simulink model "M4B11_modified_AGC_PI"  (R2025a)
settings: Solver=VariableStepAuto  StartTime=0.0  StopTime=100  RelTol=1e-3
InitFcn:
  | clear;
  | load('parameterinit.mat');
  | set_param('M4B11_modified_AGC_PI/Python2Sim','value','[0 0 0 0 0 0 0 0]');
  | acom=100;
  | bcom=50;
  | lam=100;
values from neighbouring files (symbols this model uses):
  ACgirdinit =     [datainit.mat]    (also in parameterinit.mat)
  AVm0 = [11.3576294988 11.3576294988]    [datainit.mat]    (also in parameterinit.mat)
  commun = [1 1 1 0]    [datainit.mat]    (also in initAll.m = [1,1,1,0]; parameterinit.mat)
  DataDelay = [0  0; 0  0; 0  0; 0  0]    [datainit.mat]    (also in initAll.m = 0.0*DataDelay; parameterinit.mat)
  ESinit =     [datainit.mat]    (also in parameterinit.mat)
  fB = 50    [datainit.mat]    (also in initAll.m; parameterinit.mat)
  Geninit =     [datainit.mat]    (also in initAll.m = Generator_init(opdata,SynMach_in_gidx); parameterinit.mat)
  SgridB = 100    [datainit.mat]    (also in initAll.m = resultsac.baseMVA; parameterinit.mat)
  wB = 314.159265359    [datainit.mat]    (also in initAll.m; parameterinit.mat)
  Windinit =     [datainit.mat]    (also in parameterinit.mat)
undefined symbols (not defined in the file or in its folder): c1, c2, c3, c4, c5, c6, cp_nom, lambda_nom, P_wind_base, Pelec_base, Pnom
libraries: spsBistableLib x9, slpidlib x2, simulink_extras x2
(part 1 of 6)
settings Model: Creator=LinSiQi  LastModifiedBy=86182
settings SolverCC: AlgebraicLoopSolver=TrustRegion
settings DataIOCC: DSMLogging=off  ReturnWorkspaceOutputs=off  SignalLoggingName=logout
settings DebuggingCC: UnconnectedInputMsg=warning  UnconnectedOutputMsg=warning  UnconnectedLineMsg=warning  ArithmeticOperatorsInVariantConditions=warning
settings ModelReferenceCC: EnableRefExpFcnMdlSchedulingChecks=on
settings SFSimCC: CustomCodeUndefinedFunction=UseInterfaceOnly
settings RTWCC: GPUComputeCapability=3.5  DLArmComputeVersion=19.05
settings CodeAppCC: StateflowObjectComments=on
settings SimscapeCC: SimscapeNormalizeSystem=off

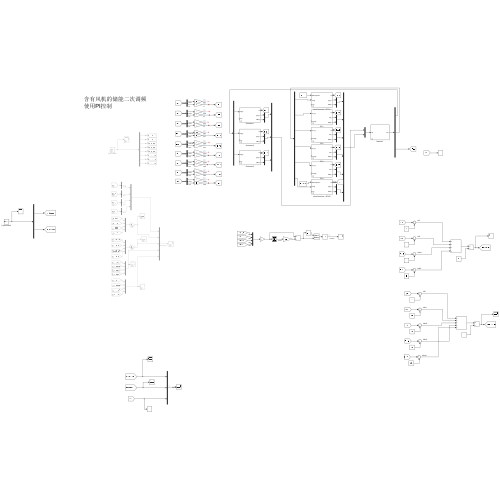
[thumbnail: Simulink's stored preview of the top-level diagram]
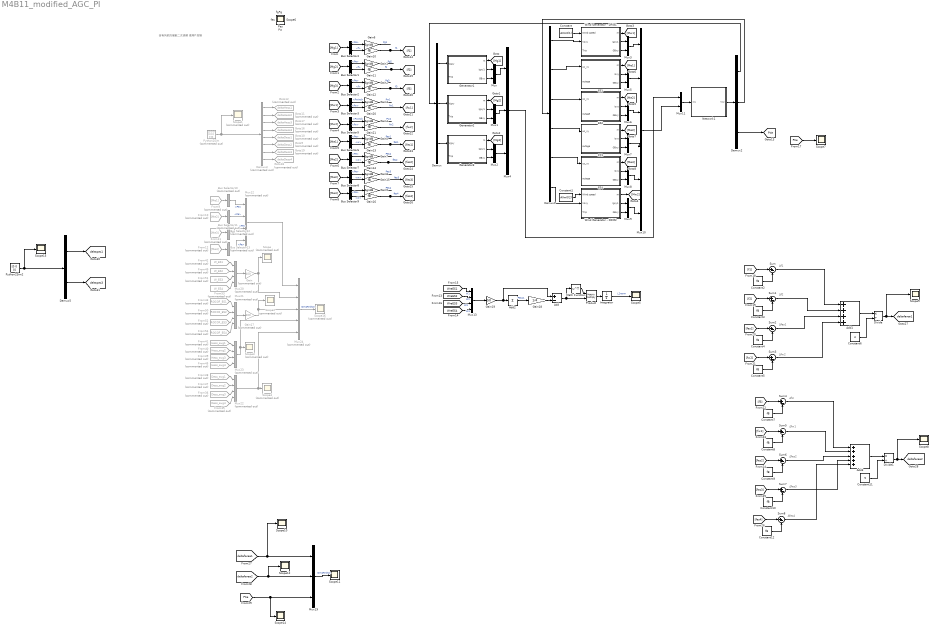
== system M4B11_modified_AGC_PI ==
  note: 含有风机的储能二次调频
      | 使用PI控制
  note: Δf1
  note: Δf2
  note: Δfes1
  note: Δfw2
  note: Δf3
  note: Δfes2
  note: Δfes3
  note: Δfw1
  note: Δfes4
  Add : Sum  Inputs=+-
  Add1 : Sum  Inputs=++++
  Add2 : Sum  Inputs=+
  Add3 : Sum  Inputs=+++++
  Bus Selector1 : BusSelector  OutputSignals=Pe,f
  Bus Selector{10..13} (4 alike) : BusSelector  Commented=on  OutputSignals=Pe
  Bus Selector2 : BusSelector  OutputSignals=Pe,f
  Bus Selector3 : BusSelector  OutputSignals=Pwind,fw
  Bus Selector4 : BusSelector  OutputSignals=Pe,f
  Bus Selector5 : BusSelector  OutputSignals=Pwind,fw
  Bus Selector{6..9} (4 alike) : BusSelector  OutputSignals=Pe,w
  Constant : Constant  Value=AVm0(1)
  Constant1 : Constant  Value=AVm0(2)
  Constant{2..5,7..10,12} (9 alike) : Constant  Value=fB
  Constant11 : Constant  Value=5
  Constant6 : Constant  Value=4
  Demux : Demux  Outputs=3
  Demux1 : Demux  Outputs=6
  Demux2 : Demux  Outputs=[6 12 1]
  Demux3 : Demux  Commented=on  Outputs=8
  Demux5 : Demux  Outputs=2
  Divide : Product  Inputs=*/
  Divide1 : Product  Inputs=*/
  ES1 : Subsystem  mask{SvscB=ESinit.SvscBi(1), SgridB=SgridB, Kppll_VSC=ESinit.Kppll(1), Kipll_VSC=ESinit.Kipll(1), Dels_hvdc=ESinit.Dels_hvdc(1), Lpr=ESinit.Lpr(1), Rpr=ESinit.Rpr(1), wB=wB, Is_xA_0=ESinit.Isx0(1), Is_yA_0=ESinit.Isy0(1), KpP_VSC_A=ESinit.KpP(1), KiP_VSC_A=ESinit.KiP(1), KpId_VSC_A=ESinit.KpId(1), KiId_VSC_A=ESinit.KiId(1), KpQ_VSC_A=ESinit.KpQ(1), KiQ_VSC_A=ESinit.KiQ(1), KpIq_VSC_A=ESinit.KpIq(1), KiIq_VSC_A=ESinit.KiIq(1), Md_A_0=ESinit.Md0(1), Mq_A_0=ESinit.Mq0(1), Nd_A_0=ESinit.Nd0(1), Nq_A_0=ESinit.Nq0(1), KIR=ESinit.Kir(1), Kdroop=ESinit.Kdroop(1), Kdistributed=ESinit.Kdistributed(1), Kdistributed_d=ESinit.Kdistributed_d(1), Kpac_VSC_A=ESinit.Kpac(1), Kiac_VSC_A=ESinit.Kiac(1), P0=ESinit.P0(1), Q0=ESinit.Q0(1), usd0=ESinit.Usd0(1)}
      mask prompts: Kppll_VSC "Kppll"; Kipll_VSC "Kipll"; KpP_VSC_A "KpP"; KiP_VSC_A "KiP"; KpId_VSC_A "KpId"; KiId_VSC_A "KiId"; KpQ_VSC_A "KpQ"; KiQ_VSC_A "KiQ"; KpIq_VSC_A "KpIq"; KiIq_VSC_A "KiIq"; Kpac_VSC_A "Kpac"; Kiac_VSC_A "Kiac"
      mask DialogControl Container48 Prompt: Base value
      mask DialogControl Container7 Prompt: PLL
      mask DialogControl Container5 Prompt: Control parameter
      mask DialogControl Container8 Prompt: inital value
      mask DialogControl Container9 Prompt: AC side
      mask DialogControl Container10 Prompt: Parameter
      mask DialogControl Container11 Prompt: Initial value
      mask DialogControl Container18 Prompt: Control parameter
      mask DialogControl Container19 Prompt: d_axis_control parameter
      mask DialogControl Container23 Prompt: d_axis_control=1
      mask DialogControl Container26 Prompt: inner current control
      mask DialogControl Container21 Prompt: q_axis_control parameter
      mask DialogControl Container29 Prompt: q_axis_control=1
      mask DialogControl Container31 Prompt: inner current control
      mask DialogControl Container22 Prompt: inital value
      mask DialogControl Container35 Prompt: outer controller
      mask DialogControl Container36 Prompt: inner control
      mask DialogControl Container27 Prompt: Inertia control
      mask DialogControl Container28 Prompt: droop control
      mask DialogControl Container300 Prompt: distributed control
      mask DialogControl Container301 Prompt: Droop distributed control
      mask DialogControl Container40 Prompt: usdq_control
      mask DialogControl Container41 Prompt: PQinitial
      mask DialogControl Container42 Prompt: usd0initial
  ES2 : Subsystem  mask{SvscB=ESinit.SvscBi(2), SgridB=SgridB, Kppll_VSC=ESinit.Kppll(2), Kipll_VSC=ESinit.Kipll(2), Dels_hvdc=ESinit.Dels_hvdc(2), Lpr=ESinit.Lpr(2), Rpr=ESinit.Rpr(2), wB=wB, Is_xA_0=ESinit.Isx0(2), Is_yA_0=ESinit.Isy0(2), KpP_VSC_A=ESinit.KpP(2), KiP_VSC_A=ESinit.KiP(2), KpId_VSC_A=ESinit.KpId(2), KiId_VSC_A=ESinit.KiId(2), KpQ_VSC_A=ESinit.KpQ(2), KiQ_VSC_A=ESinit.KiQ(2), KpIq_VSC_A=ESinit.KpIq(2), KiIq_VSC_A=ESinit.KiIq(2), Md_A_0=ESinit.Md0(2), Mq_A_0=ESinit.Mq0(2), Nd_A_0=ESinit.Nd0(2), Nq_A_0=ESinit.Nq0(2), KIR=ESinit.Kir(2), Kdroop=ESinit.Kdroop(2), Kdistributed=ESinit.Kdistributed(2), Kdistributed_d=ESinit.Kdistributed_d(2), Kpac_VSC_A=ESinit.Kpac(2), Kiac_VSC_A=ESinit.Kiac(2), P0=ESinit.P0(2), Q0=ESinit.Q0(2), usd0=ESinit.Usd0(2)}
      mask prompts: Kppll_VSC "Kppll"; Kipll_VSC "Kipll"; KpP_VSC_A "KpP"; KiP_VSC_A "KiP"; KpId_VSC_A "KpId"; KiId_VSC_A "KiId"; KpQ_VSC_A "KpQ"; KiQ_VSC_A "KiQ"; KpIq_VSC_A "KpIq"; KiIq_VSC_A "KiIq"; Kpac_VSC_A "Kpac"; Kiac_VSC_A "Kiac"
      mask DialogControl Container48 Prompt: Base value
      mask DialogControl Container7 Prompt: PLL
      mask DialogControl Container5 Prompt: Control parameter
      mask DialogControl Container8 Prompt: inital value
      mask DialogControl Container9 Prompt: AC side
      mask DialogControl Container10 Prompt: Parameter
      mask DialogControl Container11 Prompt: Initial value
      mask DialogControl Container18 Prompt: Control parameter
      mask DialogControl Container19 Prompt: d_axis_control parameter
      mask DialogControl Container23 Prompt: d_axis_control=1
      mask DialogControl Container26 Prompt: inner current control
      mask DialogControl Container21 Prompt: q_axis_control parameter
      mask DialogControl Container29 Prompt: q_axis_control=1
      mask DialogControl Container31 Prompt: inner current control
      mask DialogControl Container22 Prompt: inital value
      mask DialogControl Container35 Prompt: outer controller
      mask DialogControl Container36 Prompt: inner control
      mask DialogControl Container27 Prompt: Inertia control
      mask DialogControl Container28 Prompt: droop control
      mask DialogControl Container300 Prompt: distributed control
      mask DialogControl Container301 Prompt: Droop distributed control
      mask DialogControl Container40 Prompt: usdq_control
      mask DialogControl Container41 Prompt: PQinitial
      mask DialogControl Container42 Prompt: usd0initial
  ES3 : Subsystem  mask{SvscB=ESinit.SvscBi(3), SgridB=SgridB, Kppll_VSC=ESinit.Kppll(3), Kipll_VSC=ESinit.Kipll(3), Dels_hvdc=ESinit.Dels_hvdc(3), Lpr=ESinit.Lpr(3), Rpr=ESinit.Rpr(3), wB=wB, Is_xA_0=ESinit.Isx0(3), Is_yA_0=ESinit.Isy0(3), KpP_VSC_A=ESinit.KpP(3), KiP_VSC_A=ESinit.KiP(3), KpId_VSC_A=ESinit.KpId(3), KiId_VSC_A=ESinit.KiId(3), KpQ_VSC_A=ESinit.KpQ(3), KiQ_VSC_A=ESinit.KiQ(3), KpIq_VSC_A=ESinit.KpIq(3), KiIq_VSC_A=ESinit.KiIq(3), Md_A_0=ESinit.Md0(3), Mq_A_0=ESinit.Mq0(3), Nd_A_0=ESinit.Nd0(3), Nq_A_0=ESinit.Nq0(3), KIR=ESinit.Kir(3), Kdroop=ESinit.Kdroop(3), Kdistributed=ESinit.Kdistributed(3), Kdistributed_d=ESinit.Kdistributed_d(3), Kpac_VSC_A=ESinit.Kpac(3), Kiac_VSC_A=ESinit.Kiac(3), P0=ESinit.P0(3), Q0=ESinit.Q0(3), usd0=ESinit.Usd0(3)}
      mask prompts: Kppll_VSC "Kppll"; Kipll_VSC "Kipll"; KpP_VSC_A "KpP"; KiP_VSC_A "KiP"; KpId_VSC_A "KpId"; KiId_VSC_A "KiId"; KpQ_VSC_A "KpQ"; KiQ_VSC_A "KiQ"; KpIq_VSC_A "KpIq"; KiIq_VSC_A "KiIq"; Kpac_VSC_A "Kpac"; Kiac_VSC_A "Kiac"
      mask DialogControl Container48 Prompt: Base value
      mask DialogControl Container7 Prompt: PLL
      mask DialogControl Container5 Prompt: Control parameter
      mask DialogControl Container8 Prompt: inital value
      mask DialogControl Container9 Prompt: AC side
      mask DialogControl Container10 Prompt: Parameter
      mask DialogControl Container11 Prompt: Initial value
      mask DialogControl Container18 Prompt: Control parameter
      mask DialogControl Container19 Prompt: d_axis_control parameter
      mask DialogControl Container23 Prompt: d_axis_control=1
      mask DialogControl Container26 Prompt: inner current control
      mask DialogControl Container21 Prompt: q_axis_control parameter
      mask DialogControl Container29 Prompt: q_axis_control=1
      mask DialogControl Container31 Prompt: inner current control
      mask DialogControl Container22 Prompt: inital value
      mask DialogControl Container35 Prompt: outer controller
      mask DialogControl Container36 Prompt: inner control
      mask DialogControl Container27 Prompt: Inertia control
      mask DialogControl Container28 Prompt: droop control
      mask DialogControl Container300 Prompt: distributed control
      mask DialogControl Container301 Prompt: Droop distributed control
      mask DialogControl Container40 Prompt: usdq_control
      mask DialogControl Container41 Prompt: PQinitial
      mask DialogControl Container42 Prompt: usd0initial
  ES4 : Subsystem  mask{SvscB=ESinit.SvscBi(4), SgridB=SgridB, Kppll_VSC=ESinit.Kppll(4), Kipll_VSC=ESinit.Kipll(4), Dels_hvdc=ESinit.Dels_hvdc(4), Lpr=ESinit.Lpr(4), Rpr=ESinit.Rpr(4), wB=wB, Is_xA_0=ESinit.Isx0(4), Is_yA_0=ESinit.Isy0(4), KpP_VSC_A=ESinit.KpP(4), KiP_VSC_A=ESinit.KiP(4), KpId_VSC_A=ESinit.KpId(4), KiId_VSC_A=ESinit.KiId(4), KpQ_VSC_A=ESinit.KpQ(4), KiQ_VSC_A=ESinit.KiQ(4), KpIq_VSC_A=ESinit.KpIq(4), KiIq_VSC_A=ESinit.KiIq(4), Md_A_0=ESinit.Md0(4), Mq_A_0=ESinit.Mq0(4), Nd_A_0=ESinit.Nd0(4), Nq_A_0=ESinit.Nq0(4), KIR=ESinit.Kir(4), Kdroop=ESinit.Kdroop(4), Kdistributed=ESinit.Kdistributed(4), Kdistributed_d=ESinit.Kdistributed_d(4), Kpac_VSC_A=ESinit.Kpac(4), Kiac_VSC_A=ESinit.Kiac(4), P0=ESinit.P0(4), Q0=ESinit.Q0(4), usd0=ESinit.Usd0(4)}
      mask prompts: Kppll_VSC "Kppll"; Kipll_VSC "Kipll"; KpP_VSC_A "KpP"; KiP_VSC_A "KiP"; KpId_VSC_A "KpId"; KiId_VSC_A "KiId"; KpQ_VSC_A "KpQ"; KiQ_VSC_A "KiQ"; KpIq_VSC_A "KpIq"; KiIq_VSC_A "KiIq"; Kpac_VSC_A "Kpac"; Kiac_VSC_A "Kiac"
      mask DialogControl Container48 Prompt: Base value
      mask DialogControl Container7 Prompt: PLL
      mask DialogControl Container5 Prompt: Control parameter
      mask DialogControl Container8 Prompt: inital value
      mask DialogControl Container9 Prompt: AC side
      mask DialogControl Container10 Prompt: Parameter
      mask DialogControl Container11 Prompt: Initial value
      mask DialogControl Container18 Prompt: Control parameter
      mask DialogControl Container19 Prompt: d_axis_control parameter
      mask DialogControl Container23 Prompt: d_axis_control=1
      mask DialogControl Container26 Prompt: inner current control
      mask DialogControl Container21 Prompt: q_axis_control parameter
      mask DialogControl Container29 Prompt: q_axis_control=1
      mask DialogControl Container31 Prompt: inner current control
      mask DialogControl Container22 Prompt: inital value
      mask DialogControl Container35 Prompt: outer controller
      mask DialogControl Container36 Prompt: inner control
      mask DialogControl Container27 Prompt: Inertia control
      mask DialogControl Container28 Prompt: droop control
      mask DialogControl Container300 Prompt: distributed control
      mask DialogControl Container301 Prompt: Droop distributed control
      mask DialogControl Container40 Prompt: usdq_control
      mask DialogControl Container41 Prompt: PQinitial
      mask DialogControl Container42 Prompt: usd0initial
  From10 : From  Commented=on  GotoTag=Me2
  From11 : From  Commented=on  GotoTag=Me3
  From12 : From  Commented=on  GotoTag=Me4
  From35 : From  Commented=on  GotoTag=Dess_avg4  TagVisibility=global
  From36 : From  Commented=on  GotoTag=Dess_avg3  TagVisibility=global
  From37 : From  Commented=on  GotoTag=Dess_avg2  TagVisibility=global
  From38 : From  Commented=on  GotoTag=Dess_avg1  TagVisibility=global
  From39 : From  Commented=on  GotoTag=Hess_avg3  TagVisibility=global
  From40 : From  Commented=on  GotoTag=Hess_avg2  TagVisibility=global
  From41 : From  Commented=on  GotoTag=Hess_avg1  TagVisibility=global
  From42 : From  Commented=on  GotoTag=W_ES1  TagVisibility=global
  From43 : From  Commented=on  GotoTag=ROCOF_ES1  TagVisibility=global
  From45 : From  Commented=on  GotoTag=Hess_avg4  TagVisibility=global
  From49 : From  Commented=on  GotoTag=W_ES2  TagVisibility=global
  From50 : From  Commented=on  GotoTag=ROCOF_ES2  TagVisibility=global
  From51 : From  Commented=on  GotoTag=W_ES3  TagVisibility=global
  From52 : From  Commented=on  GotoTag=ROCOF_ES3  TagVisibility=global
  From53 : From  Commented=on  GotoTag=W_ES4  TagVisibility=global
  From54 : From  Commented=on  GotoTag=ROCOF_ES4  TagVisibility=global
  From9 : From  Commented=on  GotoTag=Me1
  Gain : Gain  Commented=on  Gain=400
  Gain{1..9} (9 alike) : Gain  Gain=SgridB
  Gain{10..16,20..21} (9 alike) : Gain  Gain=fB
  Gain17 : Gain  Commented=on  Gain=200
  Gain18 : Gain  Gain=1/4
  Gain19 : Gain  Gain=50
  Generator1 : Subsystem  mask{wB=wB, SgenB=Geninit.SgenB(1), SgridB=SgridB, Xq=Geninit.Xq(1), Xq1=Geninit.Xq1(1), Xq11=Geninit.Xq11(1), Tq0=Geninit.Tq0(1), Tq10=Geninit.Tq10(1), Eq10=Geninit.Eq1(1), Eq110=Geninit.Eq11(1), Xd=Geninit.Xd(1), Xd1=Geninit.Xd1(1), Xd11=Geninit.Xd11(1), Td0=Geninit.Td0(1), Td10=Geninit.Td10(1), Ed10=Geninit.Ed1(1), Ed110=Geninit.Ed11(1), H=Geninit.Tj(1), D=Geninit.D(1), delta0=Geninit.Delta(1), w0=1, Pm0=Geninit.Pm0(1), Ka=Geninit.Ka(1), Tb=Geninit.Tb(1), Tc=Geninit.Tc(1), Efmin=Geninit.Efmin(1), Efmax=Geninit.Efmax(1), Vref=Geninit.Vref(1), Ef10=Geninit.Vf1(1), S_PSS=Geninit.EnablePSS(1), Kpss=Geninit.kpss(1), Tw_P=Geninit.Tw_P(1), T1_P=Geninit.T1_P(1), T2_P=Geninit.T2_P(1), T3_P=Geninit.T3_P(1), T4_P=Geninit.T4_P(1), Upmax=Geninit.Upmax(1), Upmin=Geninit.Upmin(1), S_Gov=Geninit.Enablegov(1), R=Geninit.R_G(1), Ts_G=Geninit.Ts_G(1), Tc_G=Geninit.Tc_G(1), T3_G=Geninit.T3_G(1), T4_G=Geninit.T4_G(1), T5_G=Geninit.T5_G(1), dPmax=Geninit.dPmax(1), dPmin=Geninit.dPmin(1)}
      mask prompts: S_PSS "Enable PSS"; Tw_P "Tw"; T1_P "T1"; T2_P "T2"; T3_P "T3"; T4_P "T4"; S_Gov "Enable Governor"; Ts_G "Ts"; Tc_G "Tc"; T3_G "T3"; T4_G "T4"; T5_G "T5"
      mask help: This is a six-order synchronous generator with exciter system, governor and PSS.
      mask DialogControl Container6 Prompt: Machine parameter
      mask DialogControl Container25 Prompt: Base value
      mask DialogControl Container3 Prompt: q axis parameter
      mask DialogControl ParameterGroupVar Prompt: d axis parameter
      mask DialogControl Container4 Prompt: machine parameter
      mask DialogControl Container12 Prompt: Excitation System parameter
      mask DialogControl Container22 Prompt: parameter
      mask DialogControl Container23 Prompt: inital value
      mask DialogControl Container10 Prompt: PSS parameter
      mask DialogControl Container13 Prompt: Governor parameter
  Generator2 : Subsystem  mask{wB=wB, SgenB=Geninit.SgenB(2), SgridB=SgridB, Xq=Geninit.Xq(2), Xq1=Geninit.Xq1(2), Xq11=Geninit.Xq11(2), Tq0=Geninit.Tq0(2), Tq10=Geninit.Tq10(2), Eq10=Geninit.Eq1(2), Eq110=Geninit.Eq11(2), Xd=Geninit.Xd(2), Xd1=Geninit.Xd1(2), Xd11=Geninit.Xd11(2), Td0=Geninit.Td0(2), Td10=Geninit.Td10(2), Ed10=Geninit.Ed1(2), Ed110=Geninit.Ed11(2), H=Geninit.Tj(2), D=Geninit.D(2), delta0=Geninit.Delta(2), w0=1, Pm0=Geninit.Pm0(2), Ka=Geninit.Ka(2), Tb=Geninit.Tb(2), Tc=Geninit.Tc(2), Efmin=Geninit.Efmin(2), Efmax=Geninit.Efmax(2), Vref=Geninit.Vref(2), Ef10=Geninit.Vf1(2), S_PSS=Geninit.EnablePSS(2), Kpss=Geninit.kpss(2), Tw_P=Geninit.Tw_P(2), T1_P=Geninit.T1_P(2), T2_P=Geninit.T2_P(2), T3_P=Geninit.T3_P(2), T4_P=Geninit.T4_P(2), Upmax=Geninit.Upmax(2), Upmin=Geninit.Upmin(2), S_Gov=Geninit.Enablegov(2), R=Geninit.R_G(2), Ts_G=Geninit.Ts_G(2), Tc_G=Geninit.Tc_G(2), T3_G=Geninit.T3_G(2), T4_G=Geninit.T4_G(2), T5_G=Geninit.T5_G(2), dPmax=Geninit.dPmax(2), dPmin=Geninit.dPmin(2)}
      mask prompts: S_PSS "Enable PSS"; Tw_P "Tw"; T1_P "T1"; T2_P "T2"; T3_P "T3"; T4_P "T4"; S_Gov "Enable Governor"; Ts_G "Ts"; Tc_G "Tc"; T3_G "T3"; T4_G "T4"; T5_G "T5"
      mask help: This is a six-order synchronous generator with exciter system, governor and PSS.
      mask DialogControl Container6 Prompt: Machine parameter
      mask DialogControl Container25 Prompt: Base value
      mask DialogControl Container3 Prompt: q axis parameter
      mask DialogControl ParameterGroupVar Prompt: d axis parameter
      mask DialogControl Container4 Prompt: machine parameter
      mask DialogControl Container12 Prompt: Excitation System parameter
      mask DialogControl Container22 Prompt: parameter
      mask DialogControl Container23 Prompt: inital value
      mask DialogControl Container10 Prompt: PSS parameter
      mask DialogControl Container13 Prompt: Governor parameter
  Generator3 : Subsystem  mask{wB=wB, SgenB=Geninit.SgenB(3), SgridB=SgridB, Xq=Geninit.Xq(3), Xq1=Geninit.Xq1(3), Xq11=Geninit.Xq11(3), Tq0=Geninit.Tq0(3), Tq10=Geninit.Tq10(3), Eq10=Geninit.Eq1(3), Eq110=Geninit.Eq11(3), Xd=Geninit.Xd(3), Xd1=Geninit.Xd1(3), Xd11=Geninit.Xd11(3), Td0=Geninit.Td0(3), Td10=Geninit.Td10(3), Ed10=Geninit.Ed1(3), Ed110=Geninit.Ed11(3), H=Geninit.Tj(3), D=Geninit.D(3), delta0=Geninit.Delta(3), w0=1, Pm0=Geninit.Pm0(3), Ka=Geninit.Ka(3), Tb=Geninit.Tb(3), Tc=Geninit.Tc(3), Efmin=Geninit.Efmin(3), Efmax=Geninit.Efmax(3), Vref=Geninit.Vref(3), Ef10=Geninit.Vf1(3), S_PSS=Geninit.EnablePSS(3), Kpss=Geninit.kpss(3), Tw_P=Geninit.Tw_P(3), T1_P=Geninit.T1_P(3), T2_P=Geninit.T2_P(3), T3_P=Geninit.T3_P(3), T4_P=Geninit.T4_P(3), Upmax=Geninit.Upmax(3), Upmin=Geninit.Upmin(3), S_Gov=Geninit.Enablegov(3), R=Geninit.R_G(3), Ts_G=Geninit.Ts_G(3), Tc_G=Geninit.Tc_G(3), T3_G=Geninit.T3_G(3), T4_G=Geninit.T4_G(3), T5_G=Geninit.T5_G(3), dPmax=Geninit.dPmax(3), dPmin=Geninit.dPmin(3)}
      mask prompts: S_PSS "Enable PSS"; Tw_P "Tw"; T1_P "T1"; T2_P "T2"; T3_P "T3"; T4_P "T4"; S_Gov "Enable Governor"; Ts_G "Ts"; Tc_G "Tc"; T3_G "T3"; T4_G "T4"; T5_G "T5"
      mask help: This is a six-order synchronous generator with exciter system, governor and PSS.
      mask DialogControl Container6 Prompt: Machine parameter
      mask DialogControl Container25 Prompt: Base value
      mask DialogControl Container3 Prompt: q axis parameter
      mask DialogControl ParameterGroupVar Prompt: d axis parameter
      mask DialogControl Container4 Prompt: machine parameter
      mask DialogControl Container12 Prompt: Excitation System parameter
      mask DialogControl Container22 Prompt: parameter
      mask DialogControl Container23 Prompt: inital value
      mask DialogControl Container10 Prompt: PSS parameter
      mask DialogControl Container13 Prompt: Governor parameter
  Goto10 : Goto  Commented=on  GotoTag=deltaDess1  TagVisibility=global
  Goto11 : Goto  Commented=on  GotoTag=deltaHess2  TagVisibility=global
  Goto12 : Goto  Commented=on  GotoTag=deltaHess1  TagVisibility=global
  Goto16 : Goto  Commented=on  GotoTag=deltaHess4  TagVisibility=global
  Goto17 : Goto  Commented=on  GotoTag=deltaHess3  TagVisibility=global
  Goto18 : Goto  Commented=on  GotoTag=deltaDess4  TagVisibility=global
  Goto19 : Goto  Commented=on  GotoTag=deltaDess3  TagVisibility=global
  Goto9 : Goto  Commented=on  GotoTag=deltaDess2  TagVisibility=global
  Integrator : Integrator
  Math Function : Math  Operator=transpose
  Mux{,1..3,5..9,11} (10 alike) : Mux  Inputs=2
  Mux10 : Mux  Inputs=6
  Mux{12,20..23} (5 alike) : Mux  Commented=on
  Mux13 : Mux
  Mux19 : Mux  Inputs=3
  Mux24 : Mux  Commented=on  Inputs=5
  Mux4 : Mux  Inputs=3
  Network1 : Subsystem  mask{busdata=ACgirdinit.busdata{1}, linedata=ACgirdinit.linedata{1}, VSS0=ACgirdinit.VSS0{1}, LINE=ACgirdinit.fline{1}, fbus=ACgirdinit.FBUS(1), ng=ACgirdinit.ng{1}, Currentin_idx=ACgirdinit.Currentin_idx{1}, amp=ACgirdinit.amp}
  Product : Product  Multiplication=Matrix(*)
  Python2Sim : Constant  Commented=on  Value=[0 0 0 0 0 0 0 0]
  Python2Sim2 : Constant  Value=[0 0 0]
  Scope{,1..4,16} (6 alike) : Scope  Commented=on
      Scope settings: ActiveDisplayYMinimum=-0.00781  ActiveDisplayYMaximum=0.06976  DataLoggingVariableName=ScopeData7
      Scope1 settings: ActiveDisplayYMinimum=-1  ActiveDisplayYMaximum=1  DataLoggingVariableName=ScopeData5
      Scope16 settings: ActiveDisplayYMinimum=-0.65989  ActiveDisplayYMaximum=0.16966  DataLoggingVariableName=ScopeData11
      Scope2 settings: ActiveDisplayYMinimum=-2.31076  ActiveDisplayYMaximum=1.65079  DataLoggingVariableName=ScopeData8
      Scope3 settings: ActiveDisplayYMinimum=-0.04265  ActiveDisplayYMaximum=0.38387  DataLoggingVariableName=ScopeData9
      Scope4 settings: ActiveDisplayYMinimum=-1  ActiveDisplayYMaximum=1  DataLoggingVariableName=ScopeData10
  Scope{5..12,14..15} (10 alike) : Scope
      Scope10 settings: ActiveDisplayYMinimum=-0.00781  ActiveDisplayYMaximum=0.06976
      Scope11 settings: ActiveDisplayYMinimum=-0.65989  ActiveDisplayYMaximum=0.16966  DataLoggingVariableName=ScopeData2
      Scope12 settings: ActiveDisplayYMinimum=-2.31076  ActiveDisplayYMaximum=1.65079  DataLoggingVariableName=ScopeData3
      Scope14 settings: ActiveDisplayYMinimum=-1  ActiveDisplayYMaximum=1  DataLoggingVariableName=ScopeData5
      Scope15 settings: ActiveDisplayYMinimum=-1  ActiveDisplayYMaximum=1
      Scope5 settings: ActiveDisplayYMinimum=-6E-10  ActiveDisplayYMaximum=5.2E-9
      Scope7 settings: ActiveDisplayYMinimum=-0.45801744207902761  ActiveDisplayYMaximum=1.536381579384789  DataLoggingVariableName=ScopeData2
      Scope8 settings: ActiveDisplayYMinimum=-0.18612770551761812  ActiveDisplayYMaximum=0.03440492804376518  DataLoggingVariableName=ScopeData3
      Scope9 settings: ActiveDisplayYMinimum=-0.19241530083196556  ActiveDisplayYMaximum=0.037548086764144895  DataLoggingVariableName=ScopeData4
      Scope6 settings: ActiveDisplayYMinimum=49.469252933688708  ActiveDisplayYMaximum=52.493839533579845
  Sum{,1..8} (9 alike) : Sum  Inputs=|+-
  Wind Generator - DFIG1 : Subsystem  mask{NN=Windinit.NN(1), SwgBi=Windinit.SwgBi(1), SmecBi=100, SgridB=SgridB, Atheta=Windinit.Atheta(1), Kppll=Windinit.Kppll_wind(1), Kipll=Windinit.Kipll_wind(1), pitch=[500 45 2], Srotors=1.3, H=Windinit.H(1), Wr0=Windinit.Wr0(1), Xa=Windinit.Xa(1), Xa1=Windinit.Xa1(1), Lm=Windinit.Lm(1), Lr=Windinit.Lr(1), Rs=Windinit.Rs(1), Ls=Windinit.Ls(1), Ta0=Windinit.Ta0(1), NPf=Windinit.NPf(1), Za=Windinit.Za{1}, Ex0=Windinit.Ex_ref(1), Ey0=Windinit.Ey_ref(1), wB=wB, KpP_rw=Windinit.KpP_rw(1), KiP_rw=Windinit.KiP_rw(1), KpId_rw=Windinit.KpId_rw(1), KiId_rw=Windinit.KiId_rw(1), KpQ_rw=Windinit.KpQ_rw(1), KiQ_rw=Windinit.KiQ_rw(1), KpIq_rw=Windinit.KpIq_rw(1), KiIq_rw=Windinit.KiIq_rw(1), Ird_ref=Windinit.Ird_ref(1), Irq_ref=Windinit.Irq_ref(1), Qs0=Windinit.Qs0(1), KpDC_gw=Windinit.KpDC_gw(1), KiDC_gw=Windinit.KiDC_gw(1), KpId_gw=Windinit.KpId_gw(1), KiId_gw=Windinit.KiId_gw(1), KpIq_gw=Windinit.KpIq_gw(1), KiIq_gw=Windinit.KiIq_gw(1), Vdc_w=Windinit.Vdc_w(1), Icd_ref=Windinit.Icd_ref(1), Icq_ref=Windinit.Icq_ref(1), Vcd_ref=Windinit.Vcd_ref(1), Vcq_ref=Windinit.Vcq_ref(1), Lg=Windinit.Lg(1), Rg=Windinit.Rg(1), Icx0=Windinit.Icx0(1), Icy0=Windinit.Icy0(1), C_w=Windinit.C_w(1), Vdc0=Windinit.Vdc0(1)}
      mask prompts: pitch "pitch_gain，pitch_max，pitch_rate"; Srotors "Start Rotor Speed"; Ex0 "Ex"; Ey0 "Ey"
      mask init:
      | pitch_gain=pitch(1);
      | pitch_max=pitch(2);
      | pitch_rate=pitch(3);
      | 
      | %该风机模型的基准容量
      | 
      | SwgeqB=SwgBi.*NN;
      mask DialogControl Container4 Prompt: PLL/Wind turbine
      mask DialogControl Container31 Prompt: Base value
      mask DialogControl Container23 Prompt: PLL
      mask DialogControl Container6 Prompt: inital value
      mask DialogControl Container5 Prompt: PI parameter
      mask DialogControl Container24 Prompt: Wind turbine
      mask DialogControl Container25 Prompt: pitch control
      mask DialogControl Container7 Prompt: Machine parameter
      mask DialogControl Container8 Prompt: Rotor
      mask DialogControl Container9 Prompt: Machine
      mask DialogControl Container10 Prompt: parameter
      mask DialogControl Container11 Prompt: inital value
      mask DialogControl Container12 Prompt: Rotor side control
      mask DialogControl Container13 Prompt: Control parameter
      mask DialogControl Container14 Prompt: Initial value
      mask DialogControl Container15 Prompt: reactive power
      mask DialogControl Container16 Prompt: Grid side control
      mask DialogControl Container17 Prompt: parameter
      mask DialogControl Container18 Prompt: reference
      mask DialogControl Container19 Prompt: inital value
      mask DialogControl Container20 Prompt: converter function
      mask DialogControl Container21 Prompt: inital value
      mask DialogControl Container22 Prompt: DC function
  Wind Generator - DFIG2 : Subsystem  mask{NN=Windinit.NN(2), SwgBi=Windinit.SwgBi(2), SmecBi=100, SgridB=SgridB, Atheta=Windinit.Atheta(2), Kppll=Windinit.Kppll_wind(2), Kipll=Windinit.Kipll_wind(2), pitch=[500 45 2], Srotors=1.3, H=Windinit.H(2), Wr0=Windinit.Wr0(2), Xa=Windinit.Xa(2), Xa1=Windinit.Xa1(2), Lm=Windinit.Lm(2), Lr=Windinit.Lr(2), Rs=Windinit.Rs(2), Ls=Windinit.Ls(2), Ta0=Windinit.Ta0(2), NPf=Windinit.NPf(2), Za=Windinit.Za{2}, Ex0=Windinit.Ex_ref(2), Ey0=Windinit.Ey_ref(2), wB=wB, KpP_rw=Windinit.KpP_rw(2), KiP_rw=Windinit.KiP_rw(2), KpId_rw=Windinit.KpId_rw(2), KiId_rw=Windinit.KiId_rw(2), KpQ_rw=Windinit.KpQ_rw(2), KiQ_rw=Windinit.KiQ_rw(2), KpIq_rw=Windinit.KpIq_rw(2), KiIq_rw=Windinit.KiIq_rw(2), Ird_ref=Windinit.Ird_ref(2), Irq_ref=Windinit.Irq_ref(2), Qs0=Windinit.Qs0(2), KpDC_gw=Windinit.KpDC_gw(2), KiDC_gw=Windinit.KiDC_gw(2), KpId_gw=Windinit.KpId_gw(2), KiId_gw=Windinit.KiId_gw(2), KpIq_gw=Windinit.KpIq_gw(2), KiIq_gw=Windinit.KiIq_gw(2), Vdc_w=Windinit.Vdc_w(2), Icd_ref=Windinit.Icd_ref(2), Icq_ref=Windinit.Icq_ref(2), Vcd_ref=Windinit.Vcd_ref(2), Vcq_ref=Windinit.Vcq_ref(2), Lg=Windinit.Lg(2), Rg=Windinit.Rg(2), Icx0=Windinit.Icx0(2), Icy0=Windinit.Icy0(2), C_w=Windinit.C_w(2), Vdc0=Windinit.Vdc0(2)}
      mask prompts: pitch "pitch_gain，pitch_max，pitch_rate"; Srotors "Start Rotor Speed"; Ex0 "Ex"; Ey0 "Ey"
      mask init:
      | pitch_gain=pitch(1);
      | pitch_max=pitch(2);
      | pitch_rate=pitch(3);
      | 
      | %该风机模型的基准容量
      | 
      | SwgeqB=SwgBi.*NN;
      mask DialogControl Container4 Prompt: PLL/Wind turbine
      mask DialogControl Container31 Prompt: Base value
      mask DialogControl Container23 Prompt: PLL
      mask DialogControl Container6 Prompt: inital value
      mask DialogControl Container5 Prompt: PI parameter
      mask DialogControl Container24 Prompt: Wind turbine
      mask DialogControl Container25 Prompt: pitch control
      mask DialogControl Container7 Prompt: Machine parameter
      mask DialogControl Container8 Prompt: Rotor
      mask DialogControl Container9 Prompt: Machine
      mask DialogControl Container10 Prompt: parameter
      mask DialogControl Container11 Prompt: inital value
      mask DialogControl Container12 Prompt: Rotor side control
      mask DialogControl Container13 Prompt: Control parameter
      mask DialogControl Container14 Prompt: Initial value
      mask DialogControl Container15 Prompt: reactive power
      mask DialogControl Container16 Prompt: Grid side control
      mask DialogControl Container17 Prompt: parameter
      mask DialogControl Container18 Prompt: reference
      mask DialogControl Container19 Prompt: inital value
      mask DialogControl Container20 Prompt: converter function
      mask DialogControl Container21 Prompt: inital value
      mask DialogControl Container22 Prompt: DC function
  Pes : Scope
      settings: ActiveDisplayYMinimum=-216.85221612183508  ActiveDisplayYMaximum=585.021587290296  DataLoggingVariableName=ScopeData4
  Pg : Scope
      settings: ActiveDisplayYMinimum=474.29887503599929  ActiveDisplayYMaximum=889.50433221188587
  Pw : Scope
      settings: ActiveDisplayYMinimum=-13.72589  ActiveDisplayYMaximum=824.75121  DataLoggingVariableName=ScopeData3
  fes : Scope
      settings: ActiveDisplayYMinimum=49.74366180284229  ActiveDisplayYMaximum=50.030100427942727  DataLoggingVariableName=ScopeData6
  fg : Scope
      settings: ActiveDisplayYMinimum=49.768593197911578  ActiveDisplayYMaximum=50.03057306844282  DataLoggingVariableName=ScopeData2
  tag scope: Ptie=global, deltafarea1=global, deltafarea2=global, deltapes1=global, deltapes3=global
  wires:
  Mux/1 -> Mux4/1
  Generator2/2(Igxy1) -> Mux1/1
  Generator3/2(Igxy1) -> Mux2/1
  Generator1/2(Igxy1) -> Mux/1
  Generator2/3(GBxy) -> Mux1/2
  Mux1/1 -> Mux4/2
  Mux2/1 -> Mux4/3
  Generator1/3(GBxy) -> Mux/2
  Generator3/3(GBxy) -> Mux2/2
  Demux/1 -> Generator1/1(Vgxy)
  Demux/2 -> Generator2/1(Vgxy)
  Demux/3 -> Generator3/1(Vgxy)
  Constant/1 -> Wind Generator - DFIG1/1(Wind speed)
  Constant1/1 -> Wind Generator - DFIG2/1(Wind speed)
  Demux1/1 -> Wind Generator - DFIG1/2(Vsxy)
  Demux1/2 -> ES1/1(us_xy)
  Demux1/3 -> ES2/1(us_xy)
  Demux1/4 -> ES3/1(us_xy)
  Demux1/5 -> ES4/1(us_xy)
  Demux1/6 -> Wind Generator - DFIG2/2(Vsxy)
  Wind Generator - DFIG1/3(GBxy) -> Mux3/2
  Mux3/1 -> Mux10/1
  Wind Generator - DFIG1/2(Igxy1) -> Mux3/1
  ES1/3(GBxy) -> Mux5/2
  Mux5/1 -> Mux10/2
  ES1/2(isxy) -> Mux5/1
  ES2/3(GBxy) -> Mux6/2
  Mux6/1 -> Mux10/3
  ES2/2(isxy) -> Mux6/1
  ES3/3(GBxy) -> Mux7/2
  Mux7/1 -> Mux10/4
  ES3/2(isxy) -> Mux7/1
  ES4/3(GBxy) -> Mux8/2
  Mux8/1 -> Mux10/5
  ES4/2(isxy) -> Mux8/1
  Wind Generator - DFIG2/3(GBxy) -> Mux9/2
  Mux9/1 -> Mux10/6
  Wind Generator - DFIG2/2(Igxy1) -> Mux9/1
  Network1/1(Vxy) -> Demux2/1
  Demux2/1 -> Demux/1
  Demux2/2 -> Demux1/1
  Mux11/1 -> Network1/1(Ixy)
  Mux4/1 -> Mux11/1
  Mux10/1 -> Mux11/2
  Generator1/1(m) -> [Mg1]
  Generator2/1(m) -> [Mg2]
  Generator3/1(m) -> [Mg3]
  Wind Generator - DFIG1/1(m) -> [Mw1]
  Wind Generator - DFIG2/1(m) -> [Mw2]
  ES2/1(m) -> [Me2]
  ES1/1(m) -> [Me1]
  ES3/1(m) -> [Me3]
  ES4/1(m) -> [Me4]
  [Mg1] -> Bus Selector4/1
  Bus Selector4/1 -> Gain6/1  "<Pe>"
  Bus Selector1/1 -> Gain1/1  "<Pe>"
  [Mg2] -> Bus Selector1/1
  Bus Selector1/2 -> Gain11/1  "<f>"
  Bus Selector2/1 -> Gain2/1  "<Pe>"
  [Mg3] -> Bus Selector2/1
  Bus Selector2/2 -> Gain12/1  "<f>"
  [Mw1] -> Bus Selector3/1
  Bus Selector3/1 -> Gain3/1  "<Pwind>"
  [Mw2] -> Bus Selector5/1
  Bus Selector5/1 -> Gain4/1  "<Pwind>"
  [Me1] -> Bus Selector6/1
  Bus Selector6/1 -> Gain5/1  "<Pe>"
  Gain6/1 -> ?  "Pg1"
  Gain1/1 -> ?  "Pg2"
  Gain2/1 -> ?  "Pg3"
  Gain3/1 -> ?  "Pw1"
  Gain4/1 -> ?  "Pw2"
  Gain5/1 -> ?  "Pes1"
  Gain7/1 -> ?  "Pes2"
  Bus Selector7/1 -> Gain7/1  "<Pe>"
  [Me2] -> Bus Selector7/1
  [Me3] -> Bus Selector8/1
  Bus Selector8/1 -> Gain8/1  "<Pe>"
  Gain8/1 -> ?  "Pes3"
  [Me4] -> Bus Selector9/1
  Bus Selector9/1 -> Gain9/1  "<Pe>"
  Gain9/1 -> ?  "Pes4"
  Gain10/1 -> [f1]  "f1"
  Bus Selector4/2 -> Gain10/1  "<f>"
  Gain11/1 -> [f2]  "f2"
  Gain12/1 -> [f3]  "f3"
  Demux3/4 -> Goto16/1
  Demux3/5 -> Goto10/1
  Demux3/6 -> Goto9/1
  Demux3/7 -> Goto19/1
  Python2Sim/1 -> Scope1/1, Demux3/1
  Demux3/2 -> Goto11/1
  Demux3/3 -> Goto17/1
  Demux3/1 -> Goto12/1
  Demux3/8 -> Goto18/1
  Bus Selector6/2 -> Gain13/1  "<w>"
  Bus Selector7/2 -> Gain14/1  "<w>"
  Bus Selector8/2 -> Gain15/1  "<w>"
  Bus Selector9/2 -> Gain16/1  "<w>"
  Gain13/1 -> [fes1]  "fes1"
  Gain14/1 -> [fes2]  "fes2"
  Gain15/1 -> [fes3]  "fes3"
  Gain16/1 -> [fes4]  "fes4"
  From9/1 -> Bus Selector10/1
  From10/1 -> Bus Selector11/1
  From11/1 -> Bus Selector12/1
  From12/1 -> Bus Selector13/1
  Bus Selector12/1 -> Mux12/3  "<Pe>"
  Bus Selector13/1 -> Mux12/4  "<Pe>"
  Bus Selector11/1 -> Mux12/2  "<Pe>"
  Bus Selector10/1 -> Mux12/1  "<Pe>"
  From42/1 -> Mux20/1
  From51/1 -> Mux20/3
  From53/1 -> Mux20/4
  From49/1 -> Mux20/2
  Gain/1 -> Scope/1, Mux24/2
  Mux20/1 -> Gain/1
  From52/1 -> Mux21/3
  From50/1 -> Mux21/2
  From54/1 -> Mux21/4
  From43/1 -> Mux21/1
  Gain17/1 -> Scope2/1, Mux24/3
  Mux21/1 -> Gain17/1
  Mux23/1 -> Mux24/4, Scope3/1
  From45/1 -> Mux23/4
  From40/1 -> Mux23/2
  From37/1 -> Mux22/2
  From35/1 -> Mux22/4
  From36/1 -> Mux22/3
  From39/1 -> Mux23/3
  From41/1 -> Mux23/1
  From38/1 -> Mux22/1
  Mux22/1 -> Mux24/5, Scope4/1
  Mux12/1 -> Mux24/1
  Mux24/1 -> Scope16/1  "Sim2Python"
  [WreES1] -> Mux13/1  "W1"
  [WreES2] -> Mux13/2  "W2"
  [WreES3] -> Mux13/3  "W3"
  [WreES4] -> Mux13/4  "W4"
  Gain19/1 -> Add/1, Add2/1
  Add2/1 -> Gain18/1  "Pess1"
  Gain18/1 -> Add/2
  Add/1 -> Product/2, Math Function/1
  Product/1 -> Integrator/1
  Integrator/1 -> Scope5/1  "L2norm"
  Math Function/1 -> Product/1
  Mux13/1 -> Gain19/1
  Demux2/3 -> [Ptie]
  Bus Selector3/2 -> Gain20/1  "<fw>"
  Bus Selector5/2 -> Gain21/1  "<fw>"
  Gain20/1 -> [fw1]  "fw1"
  Gain21/1 -> [fw2]  "fw2"
  [Ptie] -> Scope7/1
  [f1] -> Sum/1
  Constant2/1 -> Sum/2
  [f2] -> Sum1/1
  Constant3/1 -> Sum1/2
  [fes1] -> Sum2/1
  Constant4/1 -> Sum2/2
  [fw2] -> Sum3/1
  Constant5/1 -> Sum3/2
  Sum/1 -> Add1/1
  Sum1/1 -> Add1/2
  Sum2/1 -> Add1/3
  Add1/1 -> Divide/1
  Constant6/1 -> Divide/2
  Divide1/1 -> Scope8/1, [deltafarea2]
  Add3/1 -> Divide1/1
  Constant9/1 -> Sum6/2
  Constant10/1 -> Sum7/2
  Constant8/1 -> Sum5/2
  [f3] -> Sum4/1
  Constant7/1 -> Sum4/2
  [fw1] -> Sum5/1
  Constant11/1 -> Divide1/2
  [fes3] -> Sum7/1
  [fes2] -> Sum6/1
  [fes4] -> Sum8/1
  Constant12/1 -> Sum8/2
  Divide/1 -> Scope9/1, [deltafarea1]
  Mux19/1 -> Scope11/1  "Sim2Python"
  [deltafarea1] -> Scope10/1, Mux19/1
  [deltafarea2] -> Scope12/1, Mux19/2
  [Ptie] -> Scope14/1, Mux19/3
  Python2Sim2/1 -> Scope15/1, Demux5/1
  Demux5/2 -> [deltapes3]
  Demux5/1 -> [deltapes1]
  Sum6/1 -> Add3/3
  Sum4/1 -> Add3/1
  Sum5/1 -> Add3/2
  Sum7/1 -> Add3/4
  Sum8/1 -> Add3/5
  Sum3/1 -> Add1/4

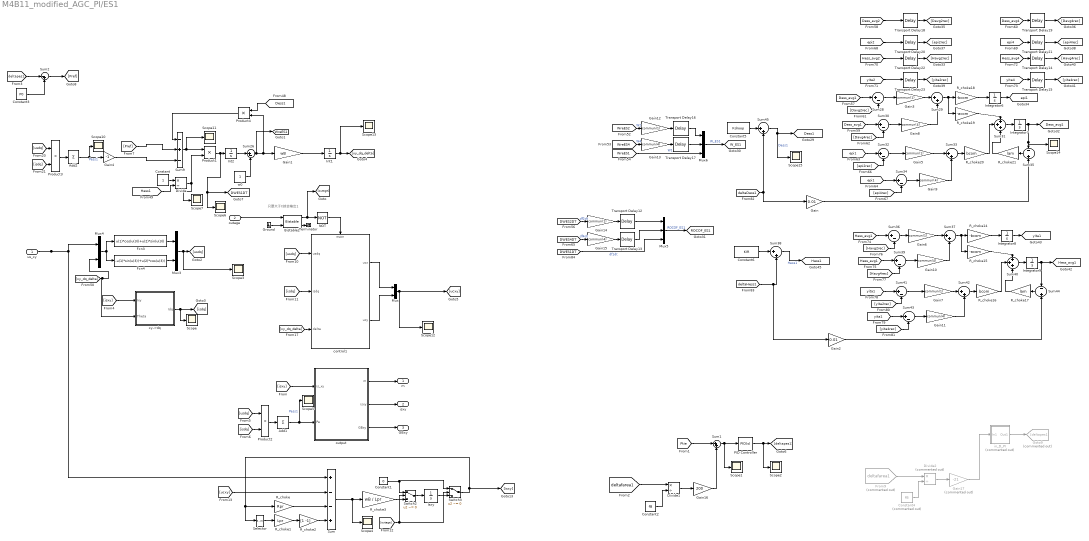
== system M4B11_modified_AGC_PI/ES1 ==
  note: 只要大于0就会输出1
  us_xy : Inport
  outage : Inport  Port=2
  " control1" : Subsystem
  Add1 : Sum  Inputs=+
  Add2 : Sum  Inputs=+
  Bistable2 : spsBistableLib/Bistable  Qpriority=Set  ic=0  Ts=0
  Constant : Constant
  Constant1 : Constant  Value=0
  Constant2 : Constant  Value=fB
  Constant3 : Constant  Value=P0
  Constant4 : Constant  Commented=on  Value=fB
  Constant5 : Constant  Value=Kdroop
  Constant6 : Constant  Value=KIR
  Divide : Product  Inputs=*/
  Divide1 : Product  Inputs=*/
  Divide2 : Product  Commented=on  Inputs=*/
  Fcn3 : Fcn  Expr=u(1)*cos(u(3))+u(2)*sin(u(3))
  Fcn4 : Fcn  Expr=-u(1)*sin(u(3))+u(2)*cos(u(3))
  From9 : From  Commented=on  GotoTag=deltafarea1  TagVisibility=global
  Gain : Gain  Gain=0.01
  Gain1 : Gain  Gain=wB  SaturateOnIntegerOverflow=on  OutDataTypeStr=Inherit: Same as input  ParamDataTypeStr=Inherit: Same as input
  Gain{8..11,13,15} (6 alike) : Gain  Gain=commun(4)
  Gain{3,5..7,12,14} (6 alike) : Gain  Gain=commun(1)
  Gain16 : Gain  Gain=200
  Gain17 : Gain  Commented=on  Gain=-21
  Gain2 : Gain  Gain=0.01
  Gain4 : Gain  Gain=-1
  Goto9 : Goto  Commented=on  GotoTag=deltapes1
  Ground : Ground
  Int1 : Integrator  InitialCondition=Dels_hvdc
  Int2 : Integrator  InitialCondition=1
  Integrator{6..9} (4 alike) : Integrator
  Isxy : Integrator  InitialCondition=[Is_xA_0 Is_yA_0]
  Mux : Mux  Inputs=2
  Mux3 : Mux  Inputs=2
  Mux4 : Mux  Inputs=2
  Mux5 : Mux  Inputs=3
  Mux6 : Mux  Inputs=3
  NOT : Logic  Operator=NOT  AllPortsSameDT=off  OutDataTypeStr=boolean
  PID Controller : slpidlib/PID Controller  Controller=PID  Form=Parallel  TimeDomain=Continuous-time  UseExternalTs=off  SampleTime=-1  IntegratorMethod=Forward Euler  FilterMethod=Forward Euler  ControllerParametersSource=internal  P=0.2  I=0.2  UseKiTs=off  D=0  UseExternalDerivativeSource=off  N=100  UseFilter=on  TunerSelectOption=Transfer Function Based (PID Tuner App)  InitialConditionSource=internal  InitialConditionForIntegrator=0  InitialConditionForFilter=0  DifferentiatorICPrevScaledInput=0  ExternalReset=none  TrackingMode=off  Kt=1  LimitOutput=off  SatLimitsSource=internal  UpperSaturationLimit=inf  LowerSaturationLimit=-inf  LinearizeAsGain=on  AntiWindupMode=none  Kb=1  LimitIntegrator=off  UpperIntegratorSaturationLimit=inf  LowerIntegratorSaturationLimit=-inf  POutMin=[]  POutMax=[]  IOutMin=[]  IOutMax=[]  DOutMin=[]  DOutMax=[]  NOutMin=[]  NOutMax=[]  SumOutMin=[]  SumOutMax=[]  SaturationOutMin=[]  SaturationOutMax=[]  PParamMin=[]  PParamMax=[]  IParamMin=[]  IParamMax=[]  DParamMin=[]  DParamMax=[]  NParamMin=[]  NParamMax=[]  KbParamMin=[]  KbParamMax=[]  KtParamMin=[]  KtParamMax=[]  KbOutMin=[]  KbOutMax=[]  KtOutMin=[]  KtOutMax=[]  IntegratorOutMin=[]  IntegratorOutMax=[]  FilterOutMin=[]  FilterOutMax=[]  SumI1OutMin=[]  SumI1OutMax=[]  SumI2OutMin=[]  SumI2OutMax=[]  SumI3OutMin=[]  SumI3OutMax=[]  SumI4OutMin=[]  SumI4OutMax=[]  SumDOutMin=[]  SumDOutMax=[]  DifferentiatorOutMin=[]  DifferentiatorOutMax=[]  FilterDiffOutCoefMin=[]  FilterDiffOutCoefMax=[]  ReciprocalOutMin=[]  ReciprocalOutMax=[]  SumDenOutMin=[]  SumDenOutMax=[]  SumNumOutMin=[]  SumNumOutMax=[]  DivideOutMin=[]  DivideOutMax=[]  UdiffTsProdOutMin=[]  UdiffTsProdOutMax=[]  NTsProdOutMin=[]  NTsProdOutMax=[]  UintegralTsProdOutMin=[]  UintegralTsProdOutMax=[]  UngainTsProdOutMin=[]  UngainTsProdOutMax=[]  ClampingZeroOutDataTypeStr=Inherit: Inherit via back propagation  ClampingZeroOutMin=[]  ClampingZeroOutMax=[]  FilterDenConstantOutDataTypeStr=Inherit: Inherit via back propagation  FilterDenConstantOutMin=[]  FilterDenConstantOutMax=[]  PCopyOutDataTypeStr=Inherit: Inherit via back propagation  PCopyOutMin=[]  PCopyOutMax=[]  NCopyOutDataTypeStr=Inherit: Inherit via back propagation  NCopyOutMin=[]  NCopyOutMax=[]  IntegratorContinuousStateAttributes=''  IntegratorStateMustResolveToSignalObject=off  IntegratorRTWStateStorageClass=Auto  FilterContinuousStateAttributes=''  FilterStateMustResolveToSignalObject=off  FilterRTWStateStorageClass=Auto  ParallelPVariant=InternalParameters  IdealPVariant=Disabled  IVariant=InternalParameters  DVariant=InternalParameters  IntegratorVariant=Continuous  SatVariant=Disabled  AWVariant=Passthrough  PCopyVariant=Disabled  TRVariant=Disabled  FdbkBlocksVariant=Forward  IdealPFdbkVariant=Disabled  SatFdbkVariant=Disabled  DerivativeFilterVariant=ContFilter  NVariant=InternalParameters  NCopyVariant=Disabled  FilterICVariant=InternalICsFilter  IntegratorICVariant=InternalICs  ExternalResetVariant=Disabled  TRSumVariant=Passthrough  SumFdbkVariant=Disabled  SumVariant=Sum_PID  TsampFilterVariant=InternalTs  TsampNgainVariant=Passthrough  TsampIntegralVariant=Disabled_SignalSpec  ExternalSaturationOutDataTypeStr=Inherit: Same as second input  DerivativeSourceVariant=ErrorSignal  PreIntVariant=InternalPreInt
  Product1 : Product
  Product2 : Product  RndMeth=Zero
  Product3 : Product  RndMeth=Zero
  Product4 : Product
  R_choke : Gain  Gain=Rpr  SaturateOnIntegerOverflow=on  OutDataTypeStr=Inherit: Same as input  ParamDataTypeStr=Inherit: Same as input
  R_choke1 : Gain  Gain=Lpr  SaturateOnIntegerOverflow=on  OutDataTypeStr=Inherit: Same as input  ParamDataTypeStr=Inherit: Same as input
  R_choke14 : Gain  Gain=-bcom  SaturateOnIntegerOverflow=on  OutDataTypeStr=Inherit: Same as input  ParamDataTypeStr=Inherit: Same as input
  R_choke15 : Gain  Gain=-acom  SaturateOnIntegerOverflow=on  OutDataTypeStr=Inherit: Same as input  ParamDataTypeStr=Inherit: Same as input
  R_choke16 : Gain  Gain=bcom  SaturateOnIntegerOverflow=on  OutDataTypeStr=Inherit: Same as input  ParamDataTypeStr=Inherit: Same as input
  R_choke17 : Gain  Gain=lam  SaturateOnIntegerOverflow=on  OutDataTypeStr=Inherit: Same as input  ParamDataTypeStr=Inherit: Same as input
  R_choke18 : Gain  Gain=-bcom  SaturateOnIntegerOverflow=on  OutDataTypeStr=Inherit: Same as input  ParamDataTypeStr=Inherit: Same as input
  R_choke19 : Gain  Gain=-acom  SaturateOnIntegerOverflow=on  OutDataTypeStr=Inherit: Same as input  ParamDataTypeStr=Inherit: Same as input
  R_choke2 : Gain  Gain=[1 -1]  SaturateOnIntegerOverflow=on  OutDataTypeStr=Inherit: Same as input  ParamDataTypeStr=Inherit: Same as input
  R_choke20 : Gain  Gain=bcom  SaturateOnIntegerOverflow=on  OutDataTypeStr=Inherit: Same as input  ParamDataTypeStr=Inherit: Same as input
  R_choke21 : Gain  Gain=lam  SaturateOnIntegerOverflow=on  OutDataTypeStr=Inherit: Same as input  ParamDataTypeStr=Inherit: Same as input
  R_choke3 : Gain  Gain=wB / Lpr  SaturateOnIntegerOverflow=on  OutDataTypeStr=Inherit: Same as input  ParamDataTypeStr=Inherit: Same as input
  Scope{,1..7,10..15} (14 alike) : Scope
      Scope settings: ActiveDisplayYMinimum=-0.0194  ActiveDisplayYMaximum=0.04689
      Scope1 settings: ActiveDisplayYMinimum=-0.49925703308591207  ActiveDisplayYMaximum=1.08481193008473  DataLoggingVariableName=ScopeData16
      Scope10 settings: ActiveDisplayYMinimum=-0.6053  ActiveDisplayYMaximum=0.06726
      Scope11 settings: ActiveDisplayYMinimum=-0.1125  ActiveDisplayYMaximum=0.0125  DataLoggingVariableName=ScopeData2
      Scope12 settings: ActiveDisplayYMinimum=0.46883  ActiveDisplayYMaximum=1.25548  DataLoggingVariableName=ScopeData3
      Scope13 settings: ActiveDisplayYMinimum=-4.33823  ActiveDisplayYMaximum=0.36599  DataLoggingVariableName=ScopeData4
      Scope14 settings: ActiveDisplayYMinimum=-0.0418  ActiveDisplayYMaximum=0.37621  DataLoggingVariableName=ScopeData2
      Scope15 settings: ActiveDisplayYMinimum=-1  ActiveDisplayYMaximum=1  DataLoggingVariableName=ScopeData3
      Scope2 settings: ActiveDisplayYMinimum=-1  ActiveDisplayYMaximum=1  DataLoggingVariableName=ScopeData17
      Scope3 settings: ActiveDisplayYMinimum=-0.14332  ActiveDisplayYMaximum=1.14443
      Scope4 settings: ActiveDisplayYMinimum=-2.8E-5  ActiveDisplayYMaximum=2.4E-5  DataLoggingVariableName=ScopeData5
      Scope5 settings: ActiveDisplayYMinimum=-0.57271  ActiveDisplayYMaximum=0.19884  DataLoggingVariableName=ScopeData7
      Scope6 settings: ActiveDisplayYMinimum=-0.00021  ActiveDisplayYMaximum=0.0004  DataLoggingVariableName=ScopeData4
      Scope7 settings: ActiveDisplayYMinimum=0.9  ActiveDisplayYMaximum=1.1  DataLoggingVariableName=ScopeData14
  Selector : Selector  InputPortWidth=2  IndexOptions=Index vector (dialog)  Indices=[2 1]  OutputSizes=1
  Sum : Sum  Inputs=+--+  SaturateOnIntegerOverflow=on
  Sum1 : Sum  Inputs=|++
  Sum2 : Sum  Inputs=|-+
  Sum{26,28,30,32,34,36,39,41,43} (9 alike) : Sum  Inputs=|+-  SaturateOnIntegerOverflow=on
  Sum{29,33,37..38,42,45} (6 alike) : Sum  Inputs=|++  SaturateOnIntegerOverflow=on
  Sum31 : Sum  Inputs=+++  SaturateOnIntegerOverflow=on
  Sum35 : Sum  Inputs=-+  SaturateOnIntegerOverflow=on
  Sum40 : Sum  Inputs=+++  SaturateOnIntegerOverflow=on
  Sum44 : Sum  Inputs=-+  SaturateOnIntegerOverflow=on
  Sum9 : Sum  Inputs=-+-  SaturateOnIntegerOverflow=on
  Switch2 : Switch  Criteria=u2 ~= 0  Threshold=0.5  InputSameDT=off
  Switch3 : Switch  Criteria=u2 ~= 0  Threshold=0.5  InputSameDT=off
  Terminator : Terminator
  Transport Delay{12,16,18,20,22..23} (6 alike) : TransportDelay  DelayTime=DataDelay(2,1)
  Transport Delay{13..15,17,19,21} (6 alike) : TransportDelay  DelayTime=DataDelay(4,2)
  in_D_PI : Subsystem  Commented=on  mask{KP_=0.1, KI_=0.1, Upper_limit=inf, Lower_limit=-inf, Upper_saturation_limit=inf, Lower_saturation_limit=-inf, integrator_init=Md_A_0}
      mask prompts: KP_ "比例系数P"; KI_ "积分系数I"; Upper_limit "限幅上限"; Lower_limit "限幅下限"; Upper_saturation_limit "积分饱和上限"; Lower_saturation_limit "积分饱和下限"; integrator_init "积分初始值"
      mask DialogControl Container4 Prompt: 控制参数
      mask DialogControl Container5 Prompt: 初始值
      mask Display: disp('PI')
  output : Subsystem
  w0 : Constant
  xy->dq : Subsystem
  m : Outport
  isxy : Outport  Port=2
  GBxy : Outport  Port=3
  tag scope: DWES1DT=global, Dess1=global, Dess_avg1=global, Hess1=global, Hess_avg1=global, ROCOF_ES1=global, W_ES1=global, WreES1=global, epi1=global, yita1=global
  wires:
  Selector/1 -> R_choke1/1
  Sum/1 -> Scope4/1, R_choke3/1
  R_choke3/1 -> Switch2/3
  Ground/1 -> Bistable2/2
  R_choke2/1 -> Sum/4
  R_choke/1 -> Sum/3
  [ucxy] -> Sum/2
  output/1(m) -> m/1
  NOT/1 -> " control1"/Enable
  R_choke1/1 -> R_choke2/1
  Bistable2/1 -> NOT/1, [outage]
  Isxy/1 -> Switch3/3
  [isxy] -> xy->dq/1(Ixy)
  [isxy] -> output/1(is_xy)
  output/2(isxy) -> isxy/1
  [xy_dq_delta] -> " control1"/3(delta)
  xy->dq/1(Idq) -> [isdq], Scope/1
  Bistable2/2 -> Terminator/1
  outage/1 -> Bistable2/1
  [outage] -> Switch2/2, Switch3/2
  [isdq] -> " control1"/2(isdq)
  " control1"/1(ucx) -> Mux/1
  Switch2/1 -> Isxy/1
  Switch3/1 -> R_choke/1, Selector/1, [isxy]
  Mux/1 -> Scope12/1, [ucxy]
  [usdq] -> " control1"/1(usdq)
  output/3(GBxy) -> GBxy/1
  Constant1/1 -> Switch2/1, Switch3/1
  " control1"/2(ucy) -> Mux/2
  [usdq] -> Product2/1
  Add1/1 -> Scope5/1, output/2(Pe)  "Pess1"
  Product2/1 -> Add1/1
  [isdq] -> Product2/2
  Product1/1 -> Scope6/1, [DWES1DT], Int2/1
  Sum26/1 -> [WreES1], Product4/2, Gain1/1
  Int2/1 -> Sum26/1
  w0/1 -> Sum26/2
  Sum9/1 -> Product1/1, Scope11/1
  Constant/1 -> Divide/1
  Divide/1 -> Product1/2, Scope7/1
  [Hess1] -> Divide/2
  us_xy/1 -> Mux4/1, Sum/1
  Fcn3/1 -> Mux3/1
  Fcn4/1 -> Mux3/2
  Mux4/1 -> Fcn3/1, Fcn4/1
  [xy_dq_delta] -> Mux4/2, xy->dq/2(Theta)
  Mux3/1 -> Scope3/1, [usdq]
  Gain4/1 -> Sum9/3
  Product4/1 -> Sum9/1
  Int1/1 -> Scope13/1, [xy_dq_delta]
  Add2/1 -> Gain4/1, Scope10/1  "Pess1"
  [usdq] -> Product3/1
  [isdq] -> Product3/2
  Product3/1 -> Add2/1
  Transport Delay19/1 -> [Davg4rec]
  R_choke20/1 -> Sum31/2
  R_choke19/1 -> Sum31/1
  [Dess_avg1] -> Sum28/1
  Transport Delay13/1 -> Mux5/2
  Transport Delay12/1 -> Mux5/1
  [Dess_avg1] -> Sum30/1
  Mux6/1 -> [W_ES1]  "W_ES1"
  [WreES1] -> Mux6/3  "W1"
  Sum38/1 -> [Hess1]  "Hess1"
  Constant5/1 -> Sum45/1
  Sum45/1 -> Scope15/1, [Dess1]  "Dess1"
  Constant6/1 -> Sum38/1
  [epi1] -> Sum34/1
  R_choke21/1 -> Sum31/3
  Integrator6/1 -> [epi1]
  Sum35/1 -> R_choke21/1
  Sum31/1 -> Integrator7/1
  Integrator7/1 -> [Dess_avg1], Scope14/1, Sum35/1
  Transport Delay21/1 -> [epi4rec]
  [epi2] -> Transport Delay20/1
  [epi4rec] -> Sum34/2
  [DWES1DT] -> Mux5/3  "df1dt"
  [Davg4rec] -> Sum30/2
  [yita2rec] -> Sum41/2
  [yita1] -> Sum41/1
  Sum40/1 -> Integrator9/1
  [deltaDess1] -> Sum45/2, Gain/1
  R_choke18/1 -> Integrator6/1
  [Havg4rec] -> Sum39/2
  [epi1] -> Sum32/1
  [Havg2rec] -> Sum36/2
  Sum42/1 -> R_choke16/1
  [Dess_avg2] -> Transport Delay18/1
  Transport Delay20/1 -> [epi2rec]
  Transport Delay14/1 -> [Havg4rec]
  [Hess_avg1] -> Sum39/1
  Mux5/1 -> [ROCOF_ES1]  "ROCOF_ES1"
  Integrator9/1 -> [Hess_avg1], Sum44/1
  Sum29/1 -> R_choke19/1, R_choke18/1
  [Davg2rec] -> Sum28/2
  [yita2] -> Transport Delay23/1
  Sum37/1 -> R_choke15/1, R_choke14/1
  R_choke14/1 -> Integrator8/1
  Integrator8/1 -> [yita1]
  Transport Delay18/1 -> [Davg2rec]
  R_choke17/1 -> Sum40/3
  Transport Delay17/1 -> Mux6/2
  R_choke15/1 -> Sum40/1
  R_choke16/1 -> Sum40/2
  [Hess_avg1] -> Sum36/1
  [deltaHess1] -> Sum38/2, Gain2/1
  Sum44/1 -> R_choke17/1
  Sum33/1 -> R_choke20/1
  Transport Delay23/1 -> [yita2rec]
  Transport Delay16/1 -> Mux6/1
  [epi2rec] -> Sum32/2
  Transport Delay22/1 -> [Havg2rec]
  Transport Delay15/1 -> [yita4rec]
  [Hess_avg2] -> Transport Delay22/1
  [Dess1] -> Product4/1
  Gain1/1 -> Int1/1
  [yita4rec] -> Sum43/2
  [yita1] -> Sum43/1
  Gain/1 -> Sum35/2
  Gain2/1 -> Sum44/2
  [Dess_avg4] -> Transport Delay19/1
  [epi4] -> Transport Delay21/1
  [Hess_avg4] -> Transport Delay14/1
  [yita4] -> Transport Delay15/1
  [WreES2] -> Gain12/1  "W2"
  Gain12/1 -> Transport Delay16/1
  [WreES4] -> Gain13/1  "W4"
  Gain13/1 -> Transport Delay17/1
  [DWES2DT] -> Gain14/1  "df2dt"
  Gain14/1 -> Transport Delay12/1
  [DWES4DT] -> Gain15/1  "df4dt"
  Gain15/1 -> Transport Delay13/1
  Gain3/1 -> Sum29/1
  Sum28/1 -> Gain3/1
  Gain5/1 -> Sum33/1
  Sum32/1 -> Gain5/1
  Sum36/1 -> Gain6/1
  Gain6/1 -> Sum37/1
  Gain7/1 -> Sum42/1
  Sum41/1 -> Gain7/1
  Sum30/1 -> Gain8/1
  Gain8/1 -> Sum29/2
  Sum34/1 -> Gain9/1
  Gain9/1 -> Sum33/2
  Sum39/1 -> Gain10/1
  Gain10/1 -> Sum37/2
  Sum43/1 -> Gain11/1
  Gain11/1 -> Sum42/2
  [Ptie] -> Sum1/1
  Gain16/1 -> Sum1/2
  Sum1/1 -> Scope1/1, PID Controller/1
  PID Controller/1 -> Scope2/1, [deltapes1]
  [deltafarea1] -> Divide1/1
  Divide1/1 -> Gain16/1
  Constant2/1 -> Divide1/2
  [deltapes1] -> Sum2/1
  Sum2/1 -> [Pref]
  Constant3/1 -> Sum2/2
  Divide2/1 -> Gain17/1
  Constant4/1 -> Divide2/2
  From9/1 -> Divide2/1
  in_D_PI/1(Out1) -> Goto9/1
  Gain17/1 -> in_D_PI/1(In1)
  [Pref] -> Sum9/2
